simulink model "PI_siulink"  (R2019a)
settings: Solver=VariableStepAuto  StartTime=0.0  StopTime=100  RelTol=1e-3
libraries: simulink x2
settings Model: Creator=Neythen  LastModifiedBy=ntreloar

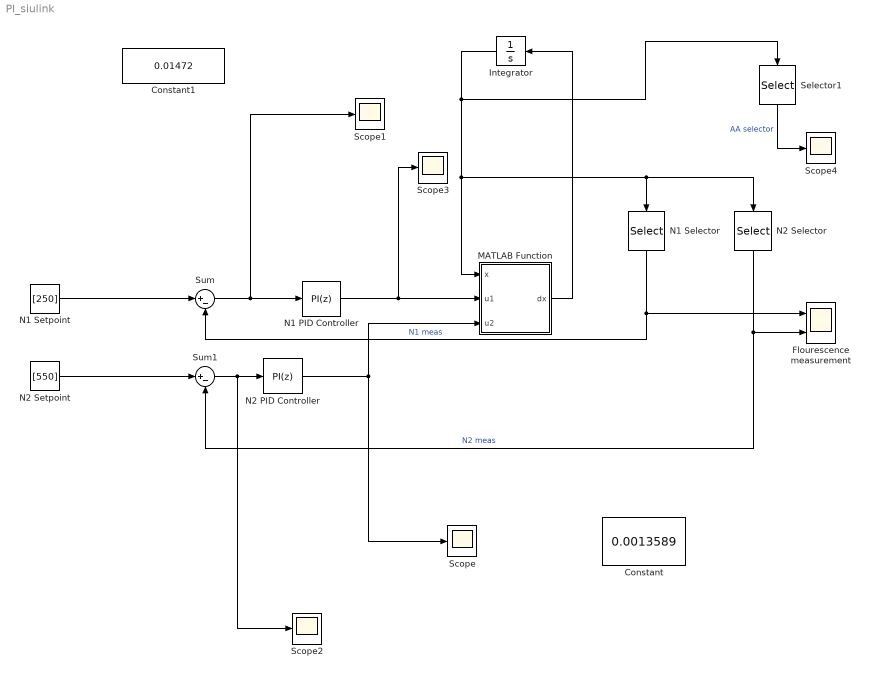
== system PI_siulink ==
  " Selector1" : Selector  InputPortWidth=5  IndexOptions=Index vector (dialog)  Indices=[3 4 ]  OutputSizes=1
  Constant : Constant  Value=0.0013589
  Constant1 : Constant  Value=0.01472
  Flourescence measurement : Scope  NumInputPorts=2
  Integrator : Integrator  InitialCondition=[250, 550, 0.01472, 0.0013589, 0.009982]'  LimitOutput=on  LowerSaturationLimit=0
  MATLAB Function : MATLAB Function  TreatAsAtomicUnit=on
  N1 Setpoint : Constant  Value=[250]
  N1 PID Controller : simulink/Continuous/PID Controller  Controller=PI  Form=Parallel  TimeDomain=Discrete-time  SampleTime=3  IntegratorMethod=Forward Euler  FilterMethod=Forward Euler  ControllerParametersSource=internal  P=0.00068642146438434  I=3.06543179141188e-05  D=0  UseFilter=on  N=100  TunerSelectOption=Transfer Function Based (PID Tuner App)  InitialConditionSource=internal  InitialConditionForIntegrator=0  InitialConditionForFilter=0  DifferentiatorICPrevScaledInput=0  ExternalReset=none  TrackingMode=off  Kt=1  LimitOutput=on  UpperSaturationLimit=inf  LowerSaturationLimit=0  LinearizeAsGain=on  AntiWindupMode=none  Kb=1  POutMin=[]  POutMax=[]  IOutMin=[]  IOutMax=[]  DOutMin=[]  DOutMax=[]  NOutMin=[]  NOutMax=[]  SumOutMin=[]  SumOutMax=[]  SaturationOutMin=[]  SaturationOutMax=[]  PParamMin=[]  PParamMax=[]  IParamMin=[]  IParamMax=[]  DParamMin=[]  DParamMax=[]  NParamMin=[]  NParamMax=[]  KbParamMin=[]  KbParamMax=[]  KtParamMin=[]  KtParamMax=[]  KbOutMin=[]  KbOutMax=[]  KtOutMin=[]  KtOutMax=[]  IntegratorOutMin=[]  IntegratorOutMax=[]  FilterOutMin=[]  FilterOutMax=[]  SumI1OutMin=[]  SumI1OutMax=[]  SumI2OutMin=[]  SumI2OutMax=[]  SumI3OutMin=[]  SumI3OutMax=[]  SumI4OutMin=[]  SumI4OutMax=[]  SumDOutMin=[]  SumDOutMax=[]  DifferentiatorOutMin=[]  DifferentiatorOutMax=[]  FilterDiffOutCoefMin=[]  FilterDiffOutCoefMax=[]  ReciprocalOutMin=[]  ReciprocalOutMax=[]  SumDenOutMin=[]  SumDenOutMax=[]  SumNumOutMin=[]  SumNumOutMax=[]  DivideOutMin=[]  DivideOutMax=[]  IntegratorContinuousStateAttributes=''  IntegratorStateMustResolveToSignalObject=off  IntegratorRTWStateStorageClass=Auto  FilterContinuousStateAttributes=''  FilterStateMustResolveToSignalObject=off  FilterRTWStateStorageClass=Auto  ParallelPVariant=InternalParameters  IdealPVariant=Disabled  IVariant=InternalParameters  DVariant=Disabled  IntegratorVariant=Discrete  SatVariant=Enabled  AWVariant=Passthrough  PCopyVariant=Disabled  TRVariant=Disabled  FdbkBlocksVariant=Forward  IdealPFdbkVariant=Disabled  SatFdbkVariant=Disabled  DerivativeFilterVariant=Disabled  NVariant=Disabled  NCopyVariant=Disabled_SignalSpec  FilterICVariant=Disabled  IntegratorICVariant=InternalICs  ExternalResetVariant=Disabled  TRSumVariant=Passthrough  SumFdbkVariant=Disabled  SumVariant=Sum_PI
  N1 Selector : Selector  InputPortWidth=5  IndexOptions=Index vector (dialog)  Indices=[1]  OutputSizes=1
  N2 Setpoint : Constant  Value=[550]
  "N2 PID Controller " : simulink/Continuous/PID Controller  Controller=PI  Form=Parallel  TimeDomain=Discrete-time  SampleTime=1/60  IntegratorMethod=Forward Euler  FilterMethod=Forward Euler  ControllerParametersSource=internal  P=0.000463861907164041  I=8.43570878573747e-06  D=0  UseFilter=on  N=100  TunerSelectOption=Transfer Function Based (PID Tuner App)  InitialConditionSource=internal  InitialConditionForIntegrator=0  InitialConditionForFilter=0  DifferentiatorICPrevScaledInput=0  ExternalReset=none  TrackingMode=off  Kt=1  LimitOutput=on  UpperSaturationLimit=inf  LowerSaturationLimit=0  LinearizeAsGain=on  AntiWindupMode=none  Kb=1  POutMin=[]  POutMax=[]  IOutMin=[]  IOutMax=[]  DOutMin=[]  DOutMax=[]  NOutMin=[]  NOutMax=[]  SumOutMin=[]  SumOutMax=[]  SaturationOutMin=[]  SaturationOutMax=[]  PParamMin=[]  PParamMax=[]  IParamMin=[]  IParamMax=[]  DParamMin=[]  DParamMax=[]  NParamMin=[]  NParamMax=[]  KbParamMin=[]  KbParamMax=[]  KtParamMin=[]  KtParamMax=[]  KbOutMin=[]  KbOutMax=[]  KtOutMin=[]  KtOutMax=[]  IntegratorOutMin=[]  IntegratorOutMax=[]  FilterOutMin=[]  FilterOutMax=[]  SumI1OutMin=[]  SumI1OutMax=[]  SumI2OutMin=[]  SumI2OutMax=[]  SumI3OutMin=[]  SumI3OutMax=[]  SumI4OutMin=[]  SumI4OutMax=[]  SumDOutMin=[]  SumDOutMax=[]  DifferentiatorOutMin=[]  DifferentiatorOutMax=[]  FilterDiffOutCoefMin=[]  FilterDiffOutCoefMax=[]  ReciprocalOutMin=[]  ReciprocalOutMax=[]  SumDenOutMin=[]  SumDenOutMax=[]  SumNumOutMin=[]  SumNumOutMax=[]  DivideOutMin=[]  DivideOutMax=[]  IntegratorContinuousStateAttributes=''  IntegratorStateMustResolveToSignalObject=off  IntegratorRTWStateStorageClass=Auto  FilterContinuousStateAttributes=''  FilterStateMustResolveToSignalObject=off  FilterRTWStateStorageClass=Auto  ParallelPVariant=InternalParameters  IdealPVariant=Disabled  IVariant=InternalParameters  DVariant=Disabled  IntegratorVariant=Discrete  SatVariant=Enabled  AWVariant=Passthrough  PCopyVariant=Disabled  TRVariant=Disabled  FdbkBlocksVariant=Forward  IdealPFdbkVariant=Disabled  SatFdbkVariant=Disabled  DerivativeFilterVariant=Disabled  NVariant=Disabled  NCopyVariant=Disabled_SignalSpec  FilterICVariant=Disabled  IntegratorICVariant=InternalICs  ExternalResetVariant=Disabled  TRSumVariant=Passthrough  SumFdbkVariant=Disabled  SumVariant=Sum_PI
  N2 Selector : Selector  InputPortWidth=5  IndexOptions=Index vector (dialog)  Indices=[2]  OutputSizes=1
  Scope{,1..4} (5 alike) : Scope
  Sum : Sum  Inputs=|+-
  Sum1 : Sum  Inputs=|+-
  wires:
  MATLAB Function/1(dx) -> Integrator/1
  Integrator/1 -> " Selector1"/1, N2 Selector/1, N1 Selector/1, MATLAB Function/1(x)
  N1 Setpoint/1 -> Sum/1
  Sum/1 -> Scope1/1, N1 PID Controller/1
  N1 Selector/1 -> Sum/2, Flourescence measurement/1  "N1 meas"
  N2 Selector/1 -> Sum1/2, Flourescence measurement/2  "N2 meas"
  N2 Setpoint/1 -> Sum1/1
  "N2 PID Controller "/1 -> Scope/1, MATLAB Function/3(u2)
  Sum1/1 -> Scope2/1, "N2 PID Controller "/1
  N1 PID Controller/1 -> MATLAB Function/2(u1), Scope3/1
  " Selector1"/1 -> Scope4/1  "AA selector"

== matlab function PI_siulink/MATLAB Function ==
  data: x input size=[5 1]; u1 input size=[1 1]; u2 input size=[1 1]; dx output size=[5 1]
function dx = derivatives(x, u1, u2)
% all derivatives exaclty the same as python implementation for the first
% step of double auxotroph
    dN = zeros(2,1);
    dC = zeros(2,1);
    dC0 = 0;
    N = zeros(2,1);
    C = zeros(2,1);
    C0 = 0;
    u = zeros(2,1);
    growth_rates = zeros(2,1);
    u(1) = u1;
    u(2) = u2;
    
    
    N = x(1:2);
    C = x(3:4);
    C0 = x(5);
   
       
    C0in = 1; q = 0.5; y = [480000., 480000.]'; y3 = [520000., 520000.]'; Rmax = [0.6, 0.6]'; Km = [0.00048776, 0.00000102115]'; Km0 = [0.00006845928, 0.00006845928]'; A = [-0.0001, -0.0001; -0.0001, -0.0001];

    growth_rates = monod_doub(C, C0, Rmax, Km, Km0);
    
    dN = N.*(growth_rates + A*N - q);
      
    dC = q.*(u - C) - (1./y).*growth_rates.*N;
  
    %disp(q.*(u - C) ); disp(- (1./y).*growth_rates.*N);
    %disp(u);disp(size(u));disp(size(C));disp(size(y));disp(size(growth_rates));disp(size(N));
       
    dC0 = q.*(C0in - C0) - sum(1./y3.*growth_rates.*N);
    
    
    dx = [dN;dC;dC0];
    
end
